simulink model "stanley"  (R2020a)
settings: Solver=FixedStepAuto  StartTime=0.0  StopTime=7  FixedStep=0.05  RelTol=1e-3
libraries: simulink x2, robotmobilelib x1, drivingvehiclecontroller x1
settings Model: Creator=Jamie  LastModifiedBy=Jamie

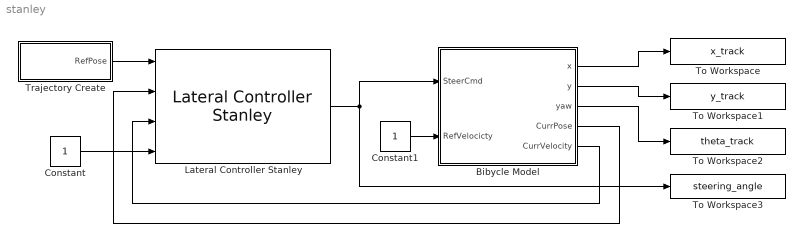
== system stanley ==
  Bibycle Model : Subsystem
  Constant : Constant
  Constant1 : Constant
  Lateral Controller Stanley : drivingvehiclecontroller/Lateral Controller Stanley  ModelType=Kinematic bicycle model  PositionGainF=5.6  PositionGainR=2.5  YawRateGain=0.2  DelayGain=0.2  VehicleMass=1575  Lf=1.2  Lr=1.6  TireStiffness=19000  Wheelbase=0.324  MaxSteeringAngle=30
      settings: SourceProductBaseCode=DR
  To Workspace : ToWorkspace  VariableName=x_track  SampleTime=-1
      settings: Save2DSignal=2-D array (concatenate along first dimension)
  To Workspace1 : ToWorkspace  VariableName=y_track  SampleTime=-1
      settings: Save2DSignal=2-D array (concatenate along first dimension)
  To Workspace2 : ToWorkspace  VariableName=theta_track  SampleTime=-1
      settings: Save2DSignal=2-D array (concatenate along first dimension)
  To Workspace3 : ToWorkspace  VariableName=steering_angle  SampleTime=-1
      settings: Save2DSignal=2-D array (concatenate along first dimension)
  Trajectory Create : Subsystem
  wires:
  Trajectory Create/1(RefPose) -> Lateral Controller Stanley/1
  Constant/1 -> Lateral Controller Stanley/4
  Lateral Controller Stanley/1 -> To Workspace3/1, Bibycle Model/1(SteerCmd)
  Bibycle Model/1(x) -> To Workspace/1
  Bibycle Model/2(y) -> To Workspace1/1
  Bibycle Model/3(yaw) -> To Workspace2/1
  Bibycle Model/4(CurrPose) -> Lateral Controller Stanley/2
  Bibycle Model/5(CurrVelocity) -> Lateral Controller Stanley/3
  Constant1/1 -> Bibycle Model/2(RefVelocicty)

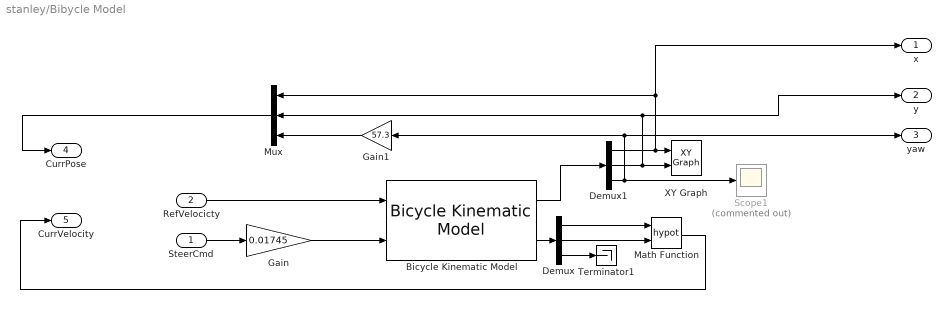
== system stanley/Bibycle Model ==
  SteerCmd : Inport
  RefVelocicty : Inport  Port=2
  Bicycle Kinematic Model : robotmobilelib/Bicycle Kinematic Model  VehicleInputs=Vehicle Speed & Steering Angle  WheelBase=0.324  VehicleSpeedRange=[-inf inf]  MaxSteeringAngle=pi/6  InitialState=[0; 0; 1.5707]  SimulateUsing=Interpreted execution
      settings: SourceProductBaseCode=RO
  Demux : Demux  Outputs=3
  Demux1 : Demux  Outputs=3
  Gain : Gain  Gain=0.01745
  Gain1 : Gain  Gain=57.3
  Math Function : Math  Operator=hypot  SaturateOnIntegerOverflow=on
  Mux : Mux  Inputs=3
  Scope1 : Scope  Commented=on
  Terminator1 : Terminator
  XY Graph : simulink/Sinks/XY Graph  xmin=-1  xmax=5  ymin=-1  ymax=5  st=-1
  x : Outport
  y : Outport  Port=2
  yaw : Outport  Port=3
  CurrPose : Outport  Port=4
  CurrVelocity : Outport  Port=5
  wires:
  Demux1/2 -> y/1, Mux/2, XY Graph/2
  Demux1/1 -> x/1, Mux/1, XY Graph/1
  Bicycle Kinematic Model/1 -> Demux1/1
  Demux/1 -> Math Function/1
  Demux1/3 -> yaw/1, Gain1/1, Scope1/1
  Bicycle Kinematic Model/2 -> Demux/1
  Math Function/1 -> CurrVelocity/1
  Gain/1 -> Bicycle Kinematic Model/2
  Demux/2 -> Math Function/2
  Demux/3 -> Terminator1/1
  RefVelocicty/1 -> Bicycle Kinematic Model/1
  Gain1/1 -> Mux/3
  Mux/1 -> CurrPose/1
  SteerCmd/1 -> Gain/1

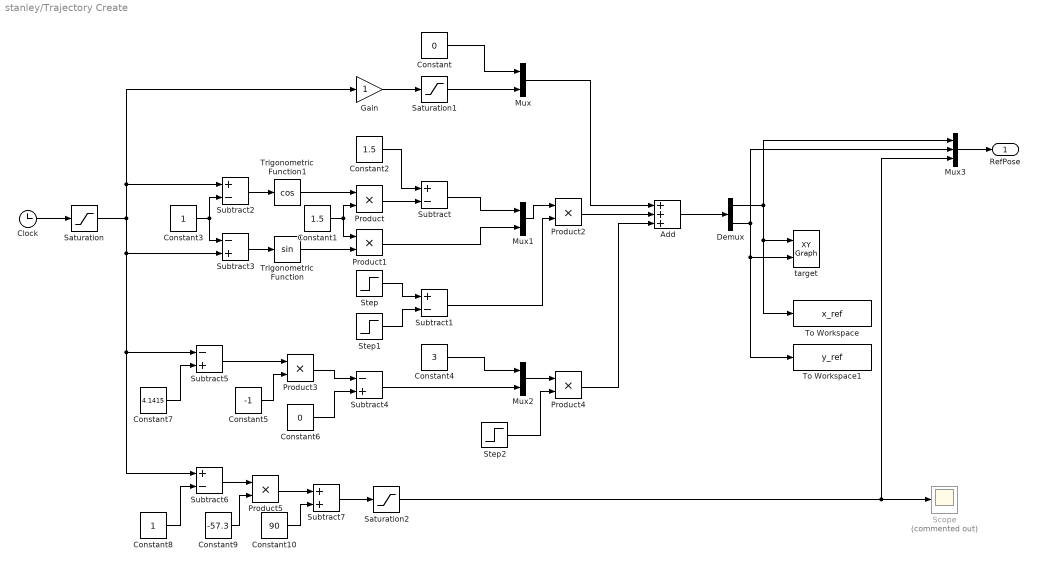
== system stanley/Trajectory Create ==
  Add : Sum  Inputs=+++
  Clock : Clock
  Constant : Constant  Value=0
  Constant1 : Constant  Value=1.5
  Constant10 : Constant  Value=90
  Constant2 : Constant  Value=1.5
  Constant3 : Constant
  Constant4 : Constant  Value=3
  Constant5 : Constant  Value=-1
  Constant6 : Constant  Value=0
  Constant7 : Constant  Value=4.1415
  Constant8 : Constant
  Constant9 : Constant  Value=-57.3
  Demux : Demux  Outputs=2
  Gain : Gain
  Mux : Mux  Inputs=2
  Mux1 : Mux  Inputs=2
  Mux2 : Mux  Inputs=2
  Mux3 : Mux  Inputs=3
  Product{,1..5} (6 alike) : Product
  Saturation : Saturate  UpperLimit=7  LowerLimit=0
  Saturation1 : Saturate  UpperLimit=1  LowerLimit=0
  Saturation2 : Saturate  UpperLimit=90  LowerLimit=-90
  Scope : Scope  Commented=on
  Step : Step  SampleTime=0
  Step1 : Step  Time=4.1415  SampleTime=0
  Step2 : Step  Time=4.1415  SampleTime=0
  Subtract{,1..2,6} (4 alike) : Sum  Inputs=+-
  Subtract3 : Sum  Inputs=-+
  Subtract4 : Sum  Inputs=-+
  Subtract5 : Sum  Inputs=-+
  Subtract7 : Sum
  To Workspace : ToWorkspace  VariableName=x_ref  SampleTime=-1
      settings: Save2DSignal=2-D array (concatenate along first dimension)
  To Workspace1 : ToWorkspace  VariableName=y_ref  SampleTime=-1
      settings: Save2DSignal=2-D array (concatenate along first dimension)
  Trigonometric Function : Trigonometry
  Trigonometric Function1 : Trigonometry  Operator=cos
  target : simulink/Sinks/XY Graph  xmin=-1  xmax=5  ymin=0  ymax=4  st=-1
  RefPose : Outport  VectorParamsAs1DForOutWhenUnconnected=off
  wires:
  Clock/1 -> Saturation/1
  Add/1 -> Demux/1
  Mux/1 -> Add/1
  Constant/1 -> Mux/1
  Saturation1/1 -> Mux/2
  Gain/1 -> Saturation1/1
  Demux/1 -> Mux3/1, To Workspace/1, target/1
  Demux/2 -> Mux3/2, To Workspace1/1, target/2
  Trigonometric Function1/1 -> Product/1
  Trigonometric Function/1 -> Product1/2
  Constant1/1 -> Product1/1, Product/2
  Product/1 -> Subtract/2
  Constant2/1 -> Subtract/1
  Subtract/1 -> Mux1/1
  Product1/1 -> Mux1/2
  Step/1 -> Subtract1/1
  Step1/1 -> Subtract1/2
  Subtract1/1 -> Product2/2
  Mux1/1 -> Product2/1
  Product2/1 -> Add/2
  Subtract2/1 -> Trigonometric Function1/1
  Subtract3/1 -> Trigonometric Function/1
  Constant3/1 -> Subtract3/1, Subtract2/2
  Constant4/1 -> Mux2/1
  Constant5/1 -> Product3/2
  Product3/1 -> Subtract4/1
  Constant6/1 -> Subtract4/2
  Subtract4/1 -> Mux2/2
  Mux2/1 -> Product4/1
  Step2/1 -> Product4/2
  Product4/1 -> Add/3
  Constant7/1 -> Subtract5/2
  Saturation/1 -> Subtract6/1, Subtract5/1, Subtract3/2, Subtract2/1, Gain/1
  Subtract5/1 -> Product3/1
  Mux3/1 -> RefPose/1
  Constant8/1 -> Subtract6/2
  Saturation2/1 -> Mux3/3, Scope/1
  Subtract6/1 -> Product5/1
  Constant9/1 -> Product5/2
  Product5/1 -> Subtract7/1
  Constant10/1 -> Subtract7/2
  Subtract7/1 -> Saturation2/1
